simulink model "park_clarke_reverse"  (R2026a)
settings: Solver=FixedStepAuto  EnableMultiTasking=on
libraries: mcbeeMathTransformLib x2
settings Model: Creator=osganig  LastModifiedBy=osganig
settings SolverCC: InitialStep=0.000001
settings HardwareCC: ProdLargestAtomicInteger=Long  ProdLargestAtomicFloat=Double  ProdHWDeviceType=ARM Compatible->ARM Cortex-M
settings RTWCC: SystemTargetFile=ert.tlc  HardwareBoard=STM32H7xx Based (Single-core)  TLCOptions=-aInlineSetEventsForThisBaseRateFcn=TLC_FALSE -aSuppressMultiTaskScheduler=TLC_FALSE -aRateBasedStepFcn=1  Toolchain=GNU Tools for STM32  BuildConfiguration=Faster Runs  DataTypeReplacement=CDataTypesFixedWidth  Description=Embedded Coder
settings ERTTargetCC: ExtModeTransport=3.0  ExtModeStaticAllocSize=2048.0  MaxIdInt64=INT64_MAX  MinIdInt64=INT64_MIN  MaxIdUint64=UINT64_MAX  MaxIdInt32=INT32_MAX  MinIdInt32=INT32_MIN  MaxIdUint32=UINT32_MAX  MaxIdInt16=INT16_MAX  MinIdInt16=INT16_MIN  MaxIdUint16=UINT16_MAX  MaxIdInt8=INT8_MAX  MinIdInt8=INT8_MIN  MaxIdUint8=UINT8_MAX  CodeReplacementLibrary=ARM Cortex-M  CodeInterfacePackaging=Reusable function  SupportNonInlinedSFcns=on

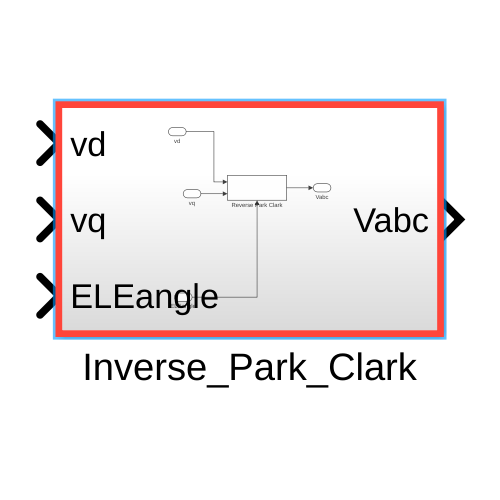
[thumbnail: Simulink's stored preview of the top-level diagram]
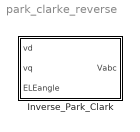
== system park_clarke_reverse ==
  Inverse_Park_Clark : Subsystem  TreatAsAtomicUnit=on  SystemSampleTime=1e-3

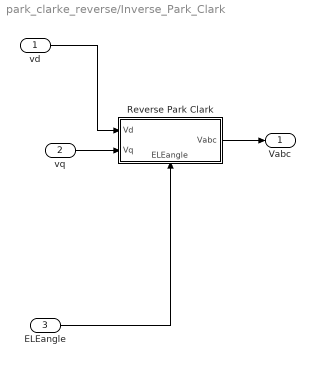
== system park_clarke_reverse/Inverse_Park_Clark ==
  vd : Inport
  vq : Inport  Port=2
  ELEangle : Inport  Port=3
  Reverse Park Clark : Subsystem
      settings: PortSchema="{\"entries\":[{\"content\":{\"sides\":[{\"content\":{\"connectorIds\":[\"In1\",\"In2\"]},\"type\":\"ConnectorPlacement.EquallySpacedRectSide\",\"uuid\":\"bb4b1d20-48ba-4b2f-b253-a250226ab501\"},{\"content\":{\"connectorIds\":[\"Out1\"],\"side\":\"RIGHT\"},\"type\":\"ConnectorPlacement.EquallySpacedRectSide\",\"uuid\":\"4768cfae-b67e-4820-9de3-2f5fe637e53a\"},{\"content\":{\"side\":\"TOP\"},\"type\":\"ConnectorPlacement.EquallySpacedRectSide\",\"uuid\":\"af639b0a-05db-45f8-bbbc-8f88455894ca\"},{\"content\":{\"connectorIds\":[\"In3\"],\"side\":\"BOTTOM\"},\"type\":\"ConnectorPlacement.EquallySpacedRectSide\",\"uuid\":\"149993ad-8fc7-43c9-baef-e4c40b0fb2ea\"}]},\"type\":\"ConnectorPlacement.EquallySpacedConnector\",\"uuid\":\"6dc62ad4-a38d-4494-a0f6-179f186f788d\"}],\"packageUris\":[\"http://schema.mathworks.com/mf0/Connector/R2020b\"],\"version\":\"1.0\"}"
  Vabc : Outport
  wires:
  vd/1 -> Reverse Park Clark/1(Vd)
  vq/1 -> Reverse Park Clark/2(Vq)
  Reverse Park Clark/1(Vabc) -> Vabc/1
  ELEangle/1 -> Reverse Park Clark/3(ELEangle)

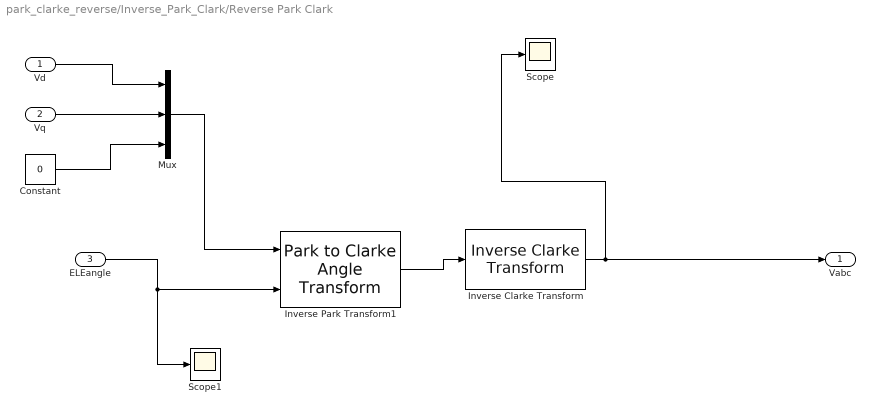
== system park_clarke_reverse/Inverse_Park_Clark/Reverse Park Clark ==
  Vd : Inport
  Vq : Inport  Port=2
  ELEangle : Inport  Port=3
  Constant : Constant  Value=0
  Inverse Clarke Transform : mcbeeMathTransformLib/Inverse Clarke Transform  PowerInvariant=off  UseWithEmbedded=on  PhaseInput=Three inputs
      settings: LibrarySourceBlock=mcblib/Controls/Math Transforms/Inverse Clarke Transform
  Inverse Park Transform1 : mcbeeMathTransformLib/Park to Clarke Angle Transform  AxisAlignment=Q-axis  UseWithEmbedded=on  PhaseInput=Three inputs  ThetaInput=Electrical position  AngleInput=Radians  N_points=1024
      settings: LibrarySourceBlock=mcblib/Controls/Math Transforms/Inverse Park Transform
  Mux : Mux  Inputs=3
  Scope : Scope
      settings: ActiveDisplayYMinimum=-233.86989625775686  ActiveDisplayYMaximum=358.80151641698012
  Scope1 : Scope
      settings: ActiveDisplayYMinimum=-11.221729676676208  ActiveDisplayYMaximum=13.302678778621274  DataLoggingVariableName=ScopeData3
  Vabc : Outport
  wires:
  Vd/1 -> Mux/1
  Vq/1 -> Mux/2
  Constant/1 -> Mux/3
  Mux/1 -> Inverse Park Transform1/1
  ELEangle/1 -> Scope1/1, Inverse Park Transform1/2
  Inverse Park Transform1/1 -> Inverse Clarke Transform/1
  Inverse Clarke Transform/1 -> Scope/1, Vabc/1
